simulink model "car"  (R2018a)
settings: Solver=VariableStepAuto  StartTime=0.0  StopTime=ttotal  RelTol=1e-3
values from neighbouring files (symbols this model uses):
  B = 15    [e_15.m]    (also in lab1.m = [5, 5, 3, 3, 20, 20])
  m = 30    [e_15.m]    (also in e_32.m = 1; e_34.m = 1; e_34b.m = 1; lab1.m = 1)
  v0 = 3    [e_15.m]    (also in lab1.m = [3, -3, 3, -3, 3, -3])
  y0 = 5    [e_15.m]    (also in lab1.m)
settings Model: Creator=root  LastModifiedBy=root

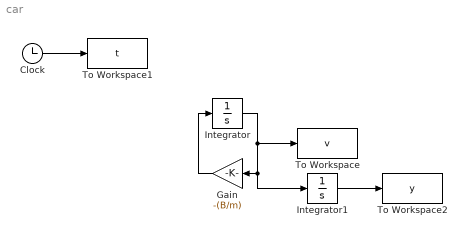
== system car ==
  Clock : Clock
  Gain : Gain  Gain=-(B/m)
  Integrator : Integrator  InitialCondition=v0
  Integrator1 : Integrator  InitialCondition=y0
  To Workspace : ToWorkspace  VariableName=v  SampleTime=-1
  To Workspace1 : ToWorkspace  VariableName=t  SampleTime=-1
  To Workspace2 : ToWorkspace  VariableName=y  SampleTime=-1
  wires:
  Integrator/1 -> Integrator1/1, Gain/1, To Workspace/1
  Gain/1 -> Integrator/1
  Clock/1 -> To Workspace1/1
  Integrator1/1 -> To Workspace2/1
